simulink model "Thesis_VehicleModel_MPC_ECMS"  (R2018b)
settings: Solver=FixedStepAuto  StartTime=0.0  StopTime=10  FixedStep=0.01  RelTol=1e-5
PostLoadFcn:
  | , if any(exist('dsrtsu_mdlpostloadfcn', 'file') == [2, 3, 6]), try dsrtsu_mdlpostloadfcn('Execute', bdroot); catch fprintf('Error in PostLoadFcn (dsrtsu_mdlpostloadfcn) for model "%s":\n %s\n', bdroot, lasterr); end, end,
InitFcn:
  | clc;clear all;
model workspace (MAT data in the model file):
  MDL : struct (value not decoded)
values from neighbouring files (symbols this model uses):
  MDL =     [MDL.mat]
libraries: simulink x14, rtican x9, autolibshared x1, mpclib x1
(part 4 of 5)

== system Thesis_VehicleModel_MPC_ECMS/Genset Powertrain Dynamics1/Rpm Controller/dSPACE CANBUS Protocol ==
  rpm cmd : Inport
  "rpm " : Inport  Port=2
  DS2202CAN_SETUP_B1_C1 : rtican/RTICAN CONTROLLER SETUP   Reserved1=[]  Reserved2=[]  Reserved3=[]  Reserved4=[]  AcceptanceMask=[]  ArbitrationField=[]  Parameters=[]  SFcnRTICANSettings=[]  MS_Struct=[]  BoardTypeNo=[]  BoardNo=[]  ChannelNo=[]  DialogFcn=[]  UnitName=[]  Revision=[]  UnitValues=[]  DSProperties=struct('RTI',struct('Version',uint32(12),'BlockType',struct('isSLSource',uint8(0),'isSLSink',uint8(0),'isHWSource',uint8(0),'isHWSink',uint8(0),'isSetup',uint8(1),'isInline',uint8(1),'isNonInline',uint8(0),'isInterrupt',uint8(0),'isChannelwise',uint8(0)),'IOBoardType','RTICAN','UnitType','NON_MESSAGE','Identifier','MASTER','DialogType','ML','BlockSet','RTICAN','SlaveProcessor','CAN'))  RTIBlockInterface=struct('InputPortsWidth',int32(0),'InputPortsActive',0,'OutputPortsWidth',int32(0),'OutputPortsActive',0,'DialogFcn','rtican_master_setup_gui','BlockDisplay',{{['CAN CONTROLLER\n SETUP'],'center'}},'IconTransparency','on','InitLevel',3,'IWork',{{{'',uint32(2)}}},'BlockName',struct('Token',{{'DS','CAN_SETUP_B','_C'}},'BlockParam',{{'BoardTypeNo','BoardNo','ChannelNo'}}),'ParameterTunableNames',{{}})  RTIBlockParameters=struct('BoardTypeNo',{{2202,'OFF',[]}},'BoardNo',{{1,'ON',[1 16]}},'ChannelNo',{{1,'ON',[1 2]}},'AcceptanceMask',{{0,'OFF',[]}},'ArbitrationField',{{0,'OFF',[]}},'Parameters',{{struct('Options',struct('DataFileSelected',1,'DataFileName',{{'dbc\dspace_test.dbc'}},'DataFileDate',{{['09-Dec-2018 18:15:36']}},'InterfaceFcn','rtican_dbc_file_parser','InterfaceFcnFileName','','AcceptanceMaskSelected',0,'NumType','hex','MaskType','STD','AcceptanceMask',0,'ArbitrationField',0,'MsgDataType','SgnSpecification','UseMultipleMessageAccess',0),'configType',1,'general',struct('Termination_common',1,'Termination_C252',1,'BusConfigurationRegister',0,'Transceiver','ISO11898','isFromLib',0),'RxReceiveStdOptions',struct('RxServiceStdEnabled',0,'RxServiceStdMsgIdent',1000,'RxServiceStdIdentNumType',1,'RxServiceStdIdentMask',0,'RxServiceStdMaskNumType',1,'RxServiceStdQueueSize',64),'RxReceiveXtdOptions',struct('RxServiceXtdEnabled',0,'RxServiceXtdMsgIdent',1001,'RxServiceXtdIdentNumType',1,'RxServiceXtdIdentMask',0,'RxServiceXtdMaskNumType',1,'RxServiceXtdQueueSize',64),'Config',struct('Baudrate',500,'SampleMode',1,'UsedParamSet',1,'isBTRvalues',0,'validSettings',1,'Advanced',struct('Baudrate',500,'Frequency',36000000,'Settings',struct('SMPL',0,'BRP',1,'NBT',18,'TSEG1',14,'TSEG2',1,'SJW',1,'SP',88),'BTR0',65,'BTR1',30)),'PartialNetworkingOptions',struct('switchedon',0,'format',1,'idmask',['XXXXX XXXXXXXX XXXXXXXX XXXXXXXX'],'idcode','0','idfilter','0','datamaskused',0,'datalength',1,'datamask','0x0000000000000000','partialnetworkenable',0)),'OFF',[]}},'CCPParameters',{{struct('CRO',struct('Format','STD','NumFormat','hex','Id',1639),'DTO',struct('Format','STD','NumFormat','hex','Id',2017),'StationAdr',struct('NumFormat','hex','Value',57),'StationId',struct('Value',['dSPACE CCP Service']),'Enabled',0),'OFF',[]}},'GroupId',{{struct('Group',{{'RTICAN'}},'No',1,'Behavior',{{'EVER'}},'BlockType',{{'SOURCE'}},'NameChangeFlag',1),'OFF',[]}},'SFcnRTICANSettings',{{struct('Baudrate',500,'configType',1,'AdvancedConfig',struct('Frequency',{},'BTR0',{},'BTR1',{}),'UsedParamSet',1,'STDMaskSelected','no','XTDMaskSelected','no','BoardType','DS2202','BoardNo',1,'ControllerNo',1,'Transceiver','ISO11898','BusConfigRegister',0,'TerminationRes',120,'UseMultipleMessageAccess','no','STDRXSrvcUsed','no','STDRXSrvcMsgId',1000,'STDRXSrvcMsgMask',0,'STDRXSrvcQueueSize',64,'XTDRXSrvcUsed','no','XTDRXSrvcMsgId',1001,'XTDRXSrvcQueueSize',64,'XTDRXSrvcMsgMask',0,'PN_IsPNTransciever',0,'PN_IsPNEnabled',0,'PN_MsgFormat',1,'PN_idcode',0,'PN_idmask',2047,'PN_datamaskused',0,'PN_datalength',0,'PN_datamask',['0xFF, 0xFF, 0xFF, 0xFF, 0xFF, 0xFF, 0xFF, 0xFF']),'OFF',[]}},'SFcnRTICCPSettings',{{struct('CRO',struct('Format','STD','NumFormat','hex','Id',1639),'DTO',struct('Format','STD','NumFormat','hex','Id',2017),'StationAdr',struct('NumFormat','hex','Value',57),'StationId',struct('Value',['dSPACE CCP Service']),'Enabled',0),'OFF',[]}},'TLCFileName',{{'rtican_master_setup','OFF',[]}},'XCPParameters',{{struct('MASTER',struct('Format','STD','NumFormat','hex','Id',256),'SLAVE',struct('Format','STD','NumFormat','hex','Id',510),'Enabled',0,'PIDTransmissionEnabled',0),'OFF',[]}},'SFcnRTIXCPSettings',{{struct('MASTER',struct('Format','STD','NumFormat','hex','Id',256),'SLAVE',struct('Format','STD','NumFormat','hex','Id',510),'Enabled',0,'PIDTransmissionEnabled',0),'OFF',[]}})  RTISFcnParameters=struct('SFcnRTICANSettings','struct','SFcnRTICCPSettings','struct','AcceptanceMask','int32','ArbitrationField','int32','TLCFileName','char','SFcnRTIXCPSettings','struct')  RTIBlockParaDefault=struct('BoardTypeNo',4302,'BoardNo',1,'ChannelNo',1,'AcceptanceMask',0,'ArbitrationField',0,'Parameters',struct('Config',{{struct('Baudrate','500','SampleMode',1,'Settings',struct('Frequency',16000000,'BTR0',64,'BTR1',28,'Baudrate',500,'ConfigStruct',struct('Baudrate',500,'Frequency',16000000,'SMPL',0,'BRP',0,'NBT',16,'TSEG1',12,'TSEG2',1,'SJW',1,'SP',87,'BTR0',64,'BTR1',28),'validSettings',1)),struct('Baudrate','500','isBTRvalues',0,'SampleMode',1,'BTR0',64,'BTR1',28,'Settings',struct('Frequency',16000000,'BTR0',128,'BTR1',103,'ListBoxItem',20,'Baudrate',500,'ConfigStruct',struct('Baudrate',500,'Frequency',16000000,'SMPL',0,'BRP',0,'NBT',16,'TSEG1',[12 12 11 11 11 10 10 10 10 9 9 9 9 8 8 8 8 7 7 7 7 6 6 6 6],'TSEG2',[1 1 2 2 2 3 3 3 3 4 4 4 4 5 5 5 5 6 6 6 6 7 7 7 7],'SJW',[0 1 0 1 2 0 1 2 3 0 1 2 3 0 1 2 3 0 1 2 3 0 1 2 3],'SP',[87 87 81 81 81 75 75 75 75 68 68 68 68 62 62 62 62 56 56 56 56 50 50 50 50],'BTR0',[0 64 0 64 128 0 64 128 192 0 64 128 192 0 64 128 192 0 64 128 192 0 64 128 192],'BTR1',[28 28 43 43 43 58 58 58 58 73 73 73 73 88 88 88 88 103 103 103 103 118 118 118 118],'StandardIndex',2),'validSettings',1))}},'Options',struct('DataFileSelected',0,'DataFileName','can_messages.dbc','DataFileDate','','InterfaceFcn','rtican_read_dbc_file','InterfaceFcnFileName','','AcceptanceMaskSelected',0,'NumType','hex','MaskType','STD','AcceptanceMask',0,'ArbitrationField',0),'configType',1,'general',struct('Termination_common',1,'Termination_C252',1,'BusConfigurationRegister',0,'Transceiver','ISO11898','isFromLib',1)),'CCPParameters',struct('CRO',struct('Format','STD','NumFormat','hex','Id',1639),'DTO',struct('Format','STD','NumFormat','hex','Id',2017),'StationAdr',struct('NumFormat','hex','Value',57),'StationId',struct('Value',['dSPACE CCP Service']),'Enabled',0),'GroupId',struct('Group',{{'RTICAN'}},'No',1,'Behavior',{{'EVER'}},'BlockType',{{'SOURCE'}},'NameChangeFlag',1),'SFcnRTICANSettings',struct('Baudrate',500,'Frequency',16000000,'BitTiming0','0x40','BitTiming1','0x1C','STDMaskSelected','no','XTDMaskSelected','no','BoardType','DS4302','BoardNo',1,'ControllerNo',1,'Transceiver','ISO11898','BusConfigRegister',0,'TerminationRes',120),'SFcnRTICCPSettings',struct('CRO',struct('Format','STD','NumFormat','hex','Id',1639),'DTO',struct('Format','STD','NumFormat','hex','Id',2017),'StationAdr',struct('NumFormat','hex','Value',57),'StationId',struct('Value',['dSPACE CCP Service']),'Enabled',0),'TLCFileName','rtican_master_setup','XCPParameters',struct('MASTER',struct('Format','STD','NumFormat','hex','Id',256),'SLAVE',struct('Format','STD','NumFormat','hex','Id',510),'Enabled',0,'PIDTransmissionEnabled',0),'SFcnRTIXCPSettings',struct('MASTER',struct('Format','STD','NumFormat','hex','Id',256),'SLAVE',struct('Format','STD','NumFormat','hex','Id',510),'Enabled',0,'PIDTransmissionEnabled',0))
      settings: AttributesFormatString=Group Id: RTICAN1\n  SourceProductName=dSPACE RTI CAN Blockset
  Data Type Conversion : DataTypeConversion  OutDataTypeStr=int16
  Data Type Conversion1 : DataTypeConversion  OutDataTypeStr=int16
  Data Type Conversion2 : DataTypeConversion  OutDataTypeStr=double
  Terminator{,1..3} (4 alike) : Terminator
  message : rtican/RTICAN Transmit (TX)   Reserved1=[]  Reserved2=[]  Reserved3=[]  Reserved4=[]  SfcnMessage=[]  Msg_Struct=[]  BoardTypeNo=[]  BoardNo=[]  ChannelNo=[]  Parameters=[]  DialogFcn=[]  UnitName=[]  Revision=[]  UnitValues=[]  DSProperties=struct('RTI',struct('Version',uint32(5),'BlockType',struct('isSLSource',uint8(1),'isSLSink',uint8(1),'isHWSource',uint8(0),'isHWSink',uint8(0),'isSetup',uint8(0),'isInline',uint8(1),'isNonInline',uint8(0),'isInterrupt',uint8(0),'isChannelwise',uint8(0)),'IOBoardType','RTICAN','UnitType','MESSAGE','Identifier','TX','DialogType','MSVC','BlockSet','RTICAN','SlaveProcessor','CAN'))  RTIBlockInterface=struct('InputPortsWidth',int32([1 1]),'InputPortsActive',[1 1],'InputPortsName',{{'Eng_rpm','Eng_rpm_Cmd'}},'OutputPortsWidth',int32([1 1]),'OutputPortsActive',[1 1],'OutputPortsName',{{['TX status'],['TX delta time']}},'DialogFcn','rtican_message_interface_gui','BlockDisplay',{{'','center'}},'IconTransparency','on','InitLevel',3,'BlockName',struct('Token',{{'message'}}),'SampleTime',{{0.01}},'TriggerPort',{{'none'}},'EnablePort',{{'none'}},'InputPortsDataType',{{'SS_INT16','SS_INT16'}})  RTIBlockParameters=struct('BoardTypeNo',{{2202,'OFF',[]}},'BoardNo',{{1,'ON',[1 16]}},'ChannelNo',{{1,'ON',[1 2]}},'Parameters',{{struct('DataFileSupport',struct('DataFileSelectedMaster',1,'DataFileSelectedLocal',1,'DataFileName','c:\users\uwecocar3\desktop\yd_thesis_dspace_model\dbc\dspace_test.dbc|','DataFileDate',['10-Dec-2018 12:52:38'],'SelectedFile','dbc\dspace_test.dbc','InterfaceFcn','rtican_dbc_file_parser'),'Options',struct('StatusSelected',1,'TimeSelected',0,'DeltaTimeSelected',1,'DelayTimeSelected',0,'TriggerPort',struct('Selected',0,'TriggerType',0),'EnablePortSelected',0,'SignalOnPortnameSelected',1,'UserCoding',struct('Selected',0,'InterfaceFile','UserEncodingFile','FcnName','UserEncodeFcn','InportSelected',0,'InportWidth',1,'OutportSelected',0,'OutportWidth',1),'TerminationMsg',struct('Selected',0,'Byte0_7','0'),'InitialMsg',struct('Selected',0,'Byte0_7','0'),'DelayTimeTXCommandSelected',0,'EncodeSetUnusedBitsToOne',0,'EnableMsgLoopback',0),'Message',struct('MsgOnBlocknameSelected',1,'MsgName','message','MsgIdFormat',0,'MsgId',16,'MsgLength',4,'NumSignals',2,'SampleTime',0.01,'StartTime',struct('Selected',0,'Value',9),'AutoRepeatTime',struct('Selected',0,'Value',0.1),'Timeout',struct('Selected',0,'Value',0.1),'DelayTime',struct('Selected',0,'Value',0.1),'Signal',struct('SgnName',{'Eng_rpm','Eng_rpm_Cmd'},'SgnStartBit',{0,16},'SgnLength',{16,16},'ByteLayout',{0,0},'Factor',{1,1},'Offset',{0,0},'SgnComment',{'',''},'SgnUnit',{'',''},'Min',{-32768,-32768},'Max',{32767,32767},'SgnType',{0,0},'SLDataType',{'SS_INT16','SS_INT16'},'DataType',{1,1},'ModeValue',{-1,-1}),'MsgIdNumFormat',0,'MsgComment',{{''}}),'Version',1.2,'general',struct('isFromLib',0)),'OFF',[]}},'GroupId',{{struct('Group',{{'RTICAN'}},'No',1,'Behavior',{{'NAMECHANGE'}},'BlockType',{{'SINK'}},'NameChangeFlag',0),'OFF',[]}},'SFcnRTICANMessage',{{struct('MsgType','TX','SFcnPortType','Scalar','MsgName','message','MsgIdFormat','STD','MsgId',16,'MsgLength',4,'NumSignals',2,'SampleTime',0.01,'StartTime',struct('Selected','no','Value',9),'AutoRepeatTime',struct('Selected','no','Value',0.1),'Timeout',struct('Selected','no','Value',0.1),'Signal',struct('SgnName',{'Eng_rpm','Eng_rpm_Cmd'},'SgnStartBit',{0,16},'SgnLength',{16,16},'ByteLayout',{['little endian'],['little endian']},'Factor',{1,1},'Offset',{0,0},'SgnType',{'standard','standard'},'SLDataType',{'SS_INT16','SS_INT16'},'DataType',{['signed int'],['signed int']},'ModeValue',{-1,-1}),'StatusSelected','yes','TimeSelected','no','DeltaTimeSelected','yes','DelayTimeSelected','no','TriggerPort',struct('Selected','no','TriggerType',0),'EnablePortSelected','no','UserCoding',struct('Selected','no','InterfaceFile','UserEncodingFile','FcnName','UserEncodeFcn','InportSelected','no','InportWidth',1,'OutportSelected','no','OutportWidth',1),'TerminationMsg',struct('Selected','no','Byte0','0x00','Byte1','0x00','Byte2','0x00','Byte3','0x00','Byte4','0x00','Byte5','0x00','Byte6','0x00','Byte7','0x00'),'InitialMsg',struct('Selected','no','Byte0','0x00','Byte1','0x00','Byte2','0x00','Byte3','0x00','Byte4','0x00','Byte5','0x00','Byte6','0x00','Byte7','0x00'),'DelayTimeTXCommandSelected','no','EncodeSetUnusedBitsToOne','no','EnableMsgLoopback','no','BoardType','DS2202','BoardNo',1,'ControllerNo',1),'OFF',[]}},'TLCFileName',{{'rtican_tx_message','OFF',[]}})  RTISFcnParameters=struct('SFcnRTICANMessage','struct','TLCFileName','char')  RTIBlockParaDefault=struct('BoardTypeNo',4302,'BoardNo',1,'ChannelNo',1,'Parameters',struct('DataFileSupport',struct('DataFileSelectedMaster',0,'DataFileSelectedLocal',0,'DataFileName','can_messages.dbc','DataFileDate',''),'Options',struct('StatusSelected',1,'TimeSelected',1,'DeltaTimeSelected',1,'DelayTimeSelected',1,'TriggerPort',struct('Selected',0,'TriggerType','rising'),'EnablePortSelected',0,'SignalOnPortnameSelected',1,'UserCoding',struct('Selected',0,'InterfaceFile','UserEncodingFile','FcnName','UserEncodeFcn','InportSelected',0,'InportWidth',1,'OutportSelected',0,'OutportWidth',1),'TerminationMsg',struct('Selected',0,'Byte0_7','0'),'InitialMsg',struct('Selected',0,'Byte0_7','0')),'Message',struct('MsgOnBlocknameSelected',0,'MsgName',['TX Message'],'MsgIdFormat',0,'MsgId',100,'MsgLength',8,'NumSignals',1,'SampleTime',-1,'StartTime',struct('Selected',0,'Value',0),'AutoRepeatTime',struct('Selected',0,'Value',0.1),'Timeout',struct('Selected',0,'Value',0.1),'DelayTime',struct('Selected',0,'Value',0.1),'Signal',struct('SgnName',['TX signal'],'SgnStartBit',0,'SgnLength',8,'SgnType',0,'ModeValue',-1,'DataType',0,'ByteLayout',0,'Factor',1,'Offset',0,'SgnComment',{{}},'SgnUnit',''),'MsgIdNumFormat',0,'MsgComment',{{''}}),'Version',1.2,'general',struct('isFromLib',1)),'GroupId',struct('Group',{{'RTICAN'}},'No',1,'Behavior',{{'NAMECHANGE'}},'BlockType',{{'SINK'}},'NameChangeFlag',0),'SFcnRTICANMessage',struct('MsgType','TX','MsgName',['TX Message'],'MsgIdFormat','STD','MsgId',100,'MsgLength',2,'NumSignals',1,'SampleTime',-1,'StartTime',struct('Selected','no','Value',0),'AutoRepeatTime',struct('Selected','no','Value',0.1),'Timeout',struct('Selected','no','Value',0.1),'DelayTime',struct('Selected','no','Value',0.1),'Signal',struct('SgnName',['TX signal'],'SgnStartBit',0,'SgnLength',8,'SgnType','standard','ModeValue',-1,'DataType',['unsigned int'],'ByteLayout',['little endian'],'Factor',1,'Offset',0),'StatusSelected','yes','TimeSelected','yes','DeltaTimeSelected','yes','DelayTimeSelected','yes','UserCoding',struct('Selected','no','InterfaceFile','UserDecodingFile','FcnName','UserDecodeFcn','InportSelected','no','InportWidth',1,'OutportSelected','no','OutportWidth',1),'TerminationMsg',struct('Selected','no','Byte0','0x00','Byte1','0x00','Byte2','0x00','Byte3','0x00','Byte4','0x00','Byte5','0x00','Byte6','0x00','Byte7','0x00'),'InitialMsg',struct('Selected','no','Byte0','0x00','Byte1','0x00','Byte2','0x00','Byte3','0x00','Byte4','0x00','Byte5','0x00','Byte6','0x00','Byte7','0x00'),'BoardType','DS4302','BoardNo',1,'ControllerNo',1,'SFcnPortType','Scalar'),'TLCFileName','rtican_tx_message')
      settings: AttributesFormatString=Group Id: RTICAN1\n  SourceProductName=dSPACE RTI CAN Blockset
  message_back : rtican/RTICAN Receive (RX)   Reserved1=[]  Reserved2=[]  Reserved3=[]  Reserved4=[]  SfcnMessage=[]  Msg_Struct=[]  BoardTypeNo=[]  BoardNo=[]  ChannelNo=[]  Parameters=[]  DialogFcn=[]  UnitName=[]  Revision=[]  UnitValues=[]  DSProperties=struct('RTI',struct('Version',uint32(5),'BlockType',struct('isSLSource',uint8(1),'isSLSink',uint8(1),'isHWSource',uint8(0),'isHWSink',uint8(0),'isSetup',uint8(0),'isInline',uint8(1),'isNonInline',uint8(0),'isInterrupt',uint8(0),'isChannelwise',uint8(0)),'IOBoardType','RTICAN','UnitType','MESSAGE','Identifier','RX','DialogType','MSVC','BlockSet','RTICAN','SlaveProcessor','CAN'))  RTIBlockInterface=struct('OutputPortsWidth',int32([1 1 1]),'OutputPortsActive',[1 1 1],'OutputPortsName',{{'ThrottleCmd',['RX status'],['RX delta time']}},'OutputPortsLabel',{{'ThrottleCmd','',''}},'OutputPortsLabelMode','ON','InputPortsWidth',int32(1),'InputPortsActive',0,'InputPortsName',{{['User inport']}},'DialogFcn','rtican_message_interface_gui','BlockDisplay',{{'','center'}},'IconTransparency','on','ParameterTunableNames',{{}},'InitLevel',3,'BlockName',struct('Token',{{'message_back'}}),'SampleTime',{{0.01}},'TriggerPort',{{'none'}},'OutputPortsDataType',{{'SS_DOUBLE','SS_DOUBLE','SS_DOUBLE'}},'EnablePort',{{'none'}})  RTIBlockParameters=struct('BoardTypeNo',{{2202,'OFF',[]}},'BoardNo',{{1,'ON',[1 16]}},'ChannelNo',{{1,'ON',[1 2]}},'Parameters',{{struct('DataFileSupport',struct('DataFileSelectedMaster',1,'DataFileSelectedLocal',1,'DataFileName','c:\users\uwecocar3\desktop\yd_thesis_dspace_model\dbc\dspace_test.dbc|','DataFileDate',{{{['10-Dec-2018 12:52:38']}}},'SelectedFile','dbc\dspace_test.dbc','InterfaceFcn','rtican_dbc_file_parser'),'Options',struct('StatusSelected',1,'TimeSelected',0,'DeltaTimeSelected',1,'BytePortSelected',0,'MessageLengthSelected',0,'TriggerPort',struct('Selected',0,'TriggerType',0),'UserCoding',struct('Selected',0,'InterfaceFile','UserDecodingFile','FcnName','UserDecodeFcn','InportSelected',0,'InportWidth',1,'OutportSelected',0,'OutportWidth',1),'EnablePortSelected',0,'SignalOnPortnameSelected',1,'UseRXService',0),'Message',struct('MsgOnBlocknameSelected',1,'MsgName','message_back','MsgIdFormat',0,'MsgId',17,'MsgLength',4,'NumSignals',1,'SampleTime',0.01,'Signal',struct('SgnName','ThrottleCmd','SgnStartBit',0,'SgnLength',16,'SgnType',0,'ModeValue',-1,'DataType',1,'ByteLayout',0,'Factor',3.052e-5,'Offset',0,'SgnComment',{{''}},'SgnUnit','','Min',-1.00007936,'Max',1.00004884,'SLDataType','SS_DOUBLE'),'MsgIdNumFormat',0,'MsgComment',{{''}}),'Version',1.2,'general',struct('isFromLib',0)),'OFF',[]}},'GroupId',{{struct('Group',{{'RTICAN'}},'No',1,'Behavior',{{'NAMECHANGE'}},'BlockType',{{'SINK'}},'NameChangeFlag',0),'OFF',[]}},'SFcnRTICANMessage',{{struct('MsgType','RX','SFcnPortType','Scalar','MsgName','message_back','MsgIdFormat','STD','MsgId',17,'MsgLength',4,'NumSignals',1,'SampleTime',0.01,'Signal',struct('SgnName','ThrottleCmd','SgnStartBit',0,'SgnLength',16,'SgnType','standard','ModeValue',-1,'DataType',['signed int'],'ByteLayout',['little endian'],'Factor',3.052e-5,'Offset',0,'SLDataType','SS_DOUBLE'),'StatusSelected','yes','TimeSelected','no','DeltaTimeSelected','yes','BytePortSelected','no','MessageLengthSelected','no','TriggerPort',struct('Selected','no','TriggerType',0),'UserCoding',struct('Selected','no','InterfaceFile','UserDecodingFile','FcnName','UserDecodeFcn','InportSelected','no','InportWidth',1,'OutportSelected','no','OutportWidth',1),'EnablePortSelected','no','UseRXService','no','BoardType','DS2202','BoardNo',1,'ControllerNo',1),'OFF',[]}},'TLCFileName',{{'rtican_rx_message','OFF',[]}})  RTISFcnParameters=struct('SFcnRTICANMessage','struct','TLCFileName','char')  RTIBlockParaDefault=struct('BoardTypeNo',4302,'BoardNo',1,'ChannelNo',1,'Parameters',struct('DataFileSupport',struct('DataFileSelectedMaster',0,'DataFileSelectedLocal',0,'DataFileName','can_messages.dbc','DataFileDate',''),'Options',struct('StatusSelected',1,'TimeSelected',1,'DeltaTimeSelected',1,'BytePortSelected',0,'MessageLengthSelected',0,'TriggerPort',struct('Selected',0,'TriggerType','rising'),'UserCoding',struct('Selected',0,'InterfaceFile','UserDecodingFile','FcnName','UserDecodeFcn','InportSelected',0,'InportWidth',1,'OutportSelected',0,'OutportWidth',1),'EnablePortSelected',0,'SignalOnPortnameSelected',1),'Message',struct('MsgOnBlocknameSelected',0,'MsgName',['RX Message'],'MsgIdFormat',0,'MsgId',100,'MsgLength',8,'NumSignals',1,'SampleTime',-1,'Signal',struct('SgnName',['RX signal'],'SgnStartBit',0,'SgnLength',8,'SgnType',0,'ModeValue',-1,'DataType',0,'ByteLayout',0,'Factor',1,'Offset',0,'SgnComment',{{}},'SgnUnit',''),'MsgIdNumFormat',0,'MsgComment',{{''}}),'Version',1.2,'general',struct('isFromLib',1)),'GroupId',struct('Group',{{'RTICAN'}},'No',1,'Behavior',{{'NAMECHANGE'}},'BlockType',{{'SINK'}},'NameChangeFlag',0),'SFcnRTICANMessage',struct('MsgType','RX','MsgName',['RX Message'],'MsgIdFormat','STD','MsgId',100,'MsgLength',8,'NumSignals',1,'SampleTime',-1,'Signal',struct('SgnName',['RX signal'],'SgnStartBit',0,'SgnLength',8,'SgnType','standard','ModeValue',-1,'DataType',['unsigned int'],'ByteLayout',['little endian'],'Factor',1,'Offset',0),'StatusSelected','yes','TimeSelected','yes','DeltaTimeSelected','yes','BytePortSelected','no','MessageLengthSelected','no','UserCoding',struct('Selected','no','InterfaceFile','UserDecodingFile','FcnName','UserDecodeFcn','InportSelected','no','InportWidth',1,'OutportSelected','no','OutportWidth',1),'BoardType','DS4302','BoardNo',1,'ControllerNo',1,'SFcnPortType','Scalar'),'TLCFileName','rtican_rx_message')
      settings: AttributesFormatString=Group Id: RTICAN1\n  SourceProductName=dSPACE RTI CAN Blockset
  ThrottleCmd : Outport
  wires:
  message_back/2 -> Terminator/1
  message_back/3 -> Terminator1/1
  message/1 -> Terminator2/1  "TX Status"
  message/2 -> Terminator3/1
  message_back/1 -> Data Type Conversion2/1  "ThrottleCmd"
  rpm cmd/1 -> Data Type Conversion1/1
  "rpm "/1 -> Data Type Conversion/1
  Data Type Conversion/1 -> message/1
  Data Type Conversion1/1 -> message/2
  Data Type Conversion2/1 -> ThrottleCmd/1

== system Thesis_VehicleModel_MPC_ECMS/Genset Powertrain Dynamics2/Battery/DP_Battery_Model ==
  Current : Inport
  Open Circuit Voltage : Inport  Port=2
  Cpa : Constant  Value=5630*6
  Cpc : Constant  Value=54277*6
  Divide : Product  Inputs=*//
  Divide1 : Product  Inputs=*/
  Divide2 : Product  Inputs=*//
  Divide3 : Product  Inputs=*/
  Gain : Gain  Gain=-1
  Gain1 : Gain  Gain=-1
  Integrator : Integrator
  Integrator1 : Integrator
  Product : Product
  "Ro " : Constant  Value=0.06
  Rpa : Constant  Value=0.00064
  Rpc : Constant  Value=0.00839
  Sum : Sum  Inputs=|++
  Sum1 : Sum  Inputs=|++
  Sum2 : Sum  Inputs=+---
  Terminal Voltage : Outport
  wires:
  Rpa/1 -> Divide/3
  Cpa/1 -> Divide1/2, Divide/2
  Sum/1 -> Integrator/1
  Product/1 -> Sum2/2
  Divide/1 -> Gain/1
  "Ro "/1 -> Product/1
  Sum2/1 -> Terminal Voltage/1
  Open Circuit Voltage/1 -> Sum2/1
  Divide1/1 -> Sum/1
  Gain/1 -> Sum/2
  Sum1/1 -> Integrator1/1
  Divide2/1 -> Gain1/1
  Divide3/1 -> Sum1/1
  Integrator/1 -> Sum2/3, Divide/1  "Upa"
  Integrator1/1 -> Sum2/4, Divide2/1  "Upc"
  Current/1 -> Product/2, Divide1/1, Divide3/1
  Cpc/1 -> Divide3/2, Divide2/2
  Rpc/1 -> Divide2/3
  Gain1/1 -> Sum1/2

== system Thesis_VehicleModel_MPC_ECMS/Genset Powertrain Dynamics2/Engine/Engine_Dynamics  ==
  "Torque_load " : Inport
  TPS Command : Inport  Port=2
  1/Shaft_Inertia : Gain  Gain=1/0.73
  Closed throttle torque : MATLAB Function  TreatAsAtomicUnit=on
  Engine rpm-torque map : Lookup_n-D  NumberOfTableDimensions=1  BreakpointsForDimension1=[0,800,1000,1500,2000,2500,3000,3500,4000,4500,5000,6500]  Table=[100,100,105,115,125,132,136,140,142,139,135,0]  InternalRulePriority=Speed  OutMin=[0]  OutMax=[150]  RndMeth=Simplest  InputSameDT=on
  Integrator : Integrator  LimitOutput=on  LowerSaturationLimit=0
  Product : Product
  Saturation2 : Saturate  UpperLimit=1  LowerLimit=0
  Sum : Sum  Inputs=+-+
  Throttle_subsystem : TransferFcn  Denominator=[0.2 1]
  rads2rpm : Gain  Gain=30/pi
  Engine torque : Outport
  Eng_rpm : Outport  Port=2
  wires:
  Throttle_subsystem/1 -> Saturation2/1
  Engine rpm-torque map/1 -> Product/2
  [Eng_rpm] -> Engine rpm-torque map/1
  TPS Command/1 -> Throttle_subsystem/1
  Product/1 -> Engine torque/1, Sum/1  "T_eng"
  Saturation2/1 -> Product/1  "TPS"
  Integrator/1 -> Closed throttle torque/1(w), rads2rpm/1
  Sum/1 -> 1/Shaft_Inertia/1
  1/Shaft_Inertia/1 -> Integrator/1
  Closed throttle torque/1(T) -> Sum/3
  rads2rpm/1 -> [Eng_rpm], Eng_rpm/1
  "Torque_load "/1 -> Sum/2  "T_load"

== system Thesis_VehicleModel_MPC_ECMS/Genset Powertrain Dynamics2/Engine/Fuel_Consumption ==
  note: Fuel Consumption
  Genset_Cmd : Inport
  Engine Torque : Inport  Port=2
  EngPwrOut(W) : Inport  Port=3
  Engine rpm : Inport  Port=4
  Add3 : Sum
  Add4 : Sum
  Detect Increase : simulink/Logic and Bit Operations/Detect Increase  vinit=0.0  OutDataTypeStr=uint8
  Divide : Product  Inputs=*/
  Engine Efficiency Map : Lookup_n-D  BreakpointsForDimension1=MDL.EngineModel.EffMapTorque  BreakpointsForDimension2=MDL.EngineModel.EffMapRPM  Table=3600/46.4./MDL.EngineModel.EffMapData  InternalRulePriority=Speed  RndMeth=Simplest  InputSameDT=on
  Gain3 : Gain  Gain=MDL.EngineModel.EngStartEnergy
  Gain4 : Gain  Gain=1/MDL.EngineModel.LHV
  Integrator2 : Integrator
  Memory : Memory
  Saturation : Saturate  UpperLimit=1  LowerLimit=0
  Fuel Consumption(g) : Outport
  wires:
  Memory/1 -> Add3/1
  Add3/1 -> Memory/1, Gain3/1
  Detect Increase/1 -> Add3/2
  Gain4/1 -> Fuel Consumption(g)/1  "Fuel Consumption"
  [GensetCmd] -> Detect Increase/1
  Add4/1 -> Gain4/1  "Energy(J)"
  Integrator2/1 -> Add4/2
  Gain3/1 -> Add4/1
  Divide/1 -> Integrator2/1  "Pwr_Eng"
  Genset_Cmd/1 -> [GensetCmd]
  Engine Torque/1 -> Engine Efficiency Map/1
  Engine rpm/1 -> Engine Efficiency Map/2
  Engine Efficiency Map/1 -> Saturation/1
  EngPwrOut(W)/1 -> Divide/1
  Saturation/1 -> Divide/2

== system Thesis_VehicleModel_MPC_ECMS/Genset Powertrain Dynamics2/Generator/Subsystem ==
  Mech_Pwr : Inport
  "Genset Cmd " : Inport  Port=2
  Add1 : Sum  Inputs=+++
  Constant2 : Constant  Value=0
  Constant3 : Constant  Value=MDL.GeneratorModel.C0
  Gain1 : Gain  Gain=MDL.GeneratorModel.C1
  Gain2 : Gain  Gain=MDL.GeneratorModel.C2
  Math Function : Math  Operator=square  SaturateOnIntegerOverflow=on
  Switch : Switch
  Pwr_Loss : Outport
  wires:
  Mech_Pwr/1 -> Math Function/1, Gain1/1
  Constant3/1 -> Switch/1
  Add1/1 -> Pwr_Loss/1
  Gain1/1 -> Add1/2
  Gain2/1 -> Add1/3
  [GensetCmd] -> Switch/2
  Switch/1 -> Add1/1
  Constant2/1 -> Switch/3
  Math Function/1 -> Gain2/1
  "Genset Cmd "/1 -> [GensetCmd]

== system Thesis_VehicleModel_MPC_ECMS/Genset Powertrain Dynamics2/Generator/Thermal Contraint ==
  MechPwrIn : Inport
  Add : Sum  Inputs=+-
  Compare To Constant : simulink/Logic and Bit Operations/Compare To Constant  relop=<=  const=3.0  OutDataTypeStr=boolean
  Constant1 : Constant  Value=MDL.GeneratorModel.ContMechPwr
  Constant2 : Constant  Value=MDL.GeneratorModel.ContMechPwr
  Constant3 : Constant  Value=MDL.GeneratorModel.PeakMechPwr
  Gain : Gain  Gain=1/(MDL.GeneratorModel.PeakMechPwr-MDL.GeneratorModel.ContMechPwr)
  Gain1 : Gain  Gain=1/60
  Integrator : Integrator  LimitOutput=on  UpperSaturationLimit=1  LowerSaturationLimit=0
  Switch1 : Switch  Criteria=u2 ~= 0
  MaxMechPwr : Outport
  wires:
  MechPwrIn/1 -> Add/1
  Constant2/1 -> Add/2
  Add/1 -> Gain/1
  Gain/1 -> Gain1/1
  Gain1/1 -> Integrator/1
  Integrator/1 -> Compare To Constant/1
  Compare To Constant/1 -> Switch1/2
  Constant1/1 -> Switch1/1
  Constant3/1 -> Switch1/3
  Switch1/1 -> MaxMechPwr/1

== system Thesis_VehicleModel_MPC_ECMS/Genset Powertrain Dynamics2/Rpm Controller/Calculate Fix Point ==
  rpm set point : Inport
  Constant1 : Constant  Value=0
  Mux : Mux  Inputs=2
  Saturation : Saturate  UpperLimit=6000  LowerLimit=0
  rpm2rads : Gain  Gain=pi/30
  rpm_cmd : Outport
  fix point (2 states) : Outport  Port=2
  wires:
  Constant1/1 -> Mux/2
  Mux/1 -> rpm2rads/1
  rpm set point/1 -> Saturation/1
  Saturation/1 -> Mux/1, rpm_cmd/1
  rpm2rads/1 -> fix point (2 states)/1

== system Thesis_VehicleModel_MPC_ECMS/Genset Powertrain Dynamics2/Rpm Controller/Kalman Filter ==
  y : Inport
  "rpm " : Inport  Port=2
  u : Inport  Port=3
  Bu : MATLAB Function  TreatAsAtomicUnit=on
  Engine rpm-torque map : Lookup_n-D  NumberOfTableDimensions=1  BreakpointsForDimension1=[800,1000,1500,2000,2500,3000,3500,4000,4500,5000,6500]  Table=[100,105,115,125,132,136,140,142,139,135,0]  InternalRulePriority=Speed  RndMeth=Simplest  InputSameDT=on
  Gain : Gain  Gain=MDL.ThrottleController.KFL  Multiplication=Matrix(K*u)
  Gain2 : Gain  Gain=MDL.ThrottleController.KFA  Multiplication=Matrix(K*u)
  Gain4 : Gain  Gain=MDL.ThrottleController.KFC  Multiplication=Matrix(K*u)
  Integrator : Integrator
  Sum1 : Sum  Inputs=|+++
  Sum2 : Sum  Inputs=|+-
  "x_hat " : Outport
  wires:
  Sum1/1 -> Integrator/1
  Gain4/1 -> Sum2/2
  Gain/1 -> Sum1/2
  Integrator/1 -> Gain4/1, Gain2/1, "x_hat "/1
  Bu/1(y) -> Sum1/1
  Gain2/1 -> Sum1/3
  Sum2/1 -> Gain/1
  y/1 -> Sum2/1
  u/1 -> Bu/1(u)
  "rpm "/1 -> Engine rpm-torque map/1
  Engine rpm-torque map/1 -> Bu/2(Tmax)
